simulink model "buck"  (R2023b)
settings: Solver=VariableStepAuto  StartTime=0.0  StopTime=0.05  FixedStep=60e-6  MaxStep=1e-6  RelTol=1e-3
undefined symbols (not defined in the file): C, L, R, R1, R2, R3, R4, R_in, Vi
settings Model: Creator=Jackson  LastModifiedBy=Jackson

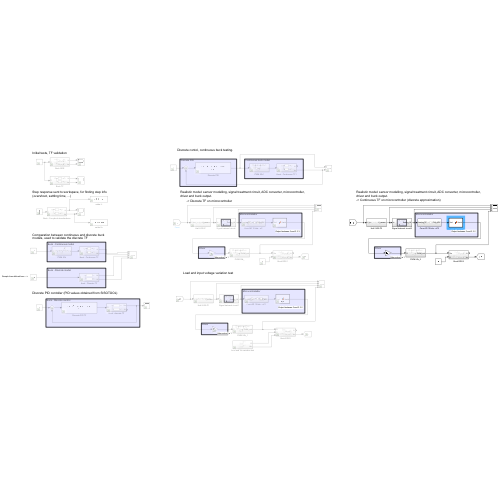
[thumbnail: Simulink's stored preview of the top-level diagram]
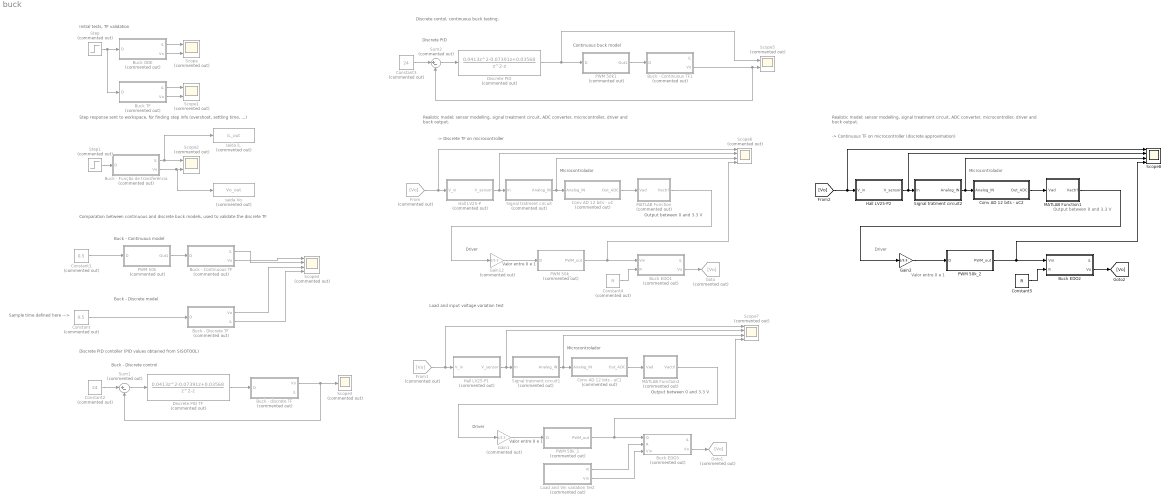
== system buck ==
  note: -> Discrete TF on microcontroller
  note: Initial tests, TF validation
  note: Output between 0 and 3.3 V
  note: Buck - Discrete control
  note: Buck - Discrete model
  note: Buck - Continuous model
  note: Discrete PID
  note: Continuous buck model
  note: Driver
  note: Microcontrolador
  note: Valor entre 0 e 1
  note: Step response sent to workspace, for finding step info (overshoot, settling time, ...)
  note: Comparation between continuous and discrete buck models, used to validate the discrete TF
  note: Sample time defined here --->
  note: Discrete PID contoller (PID values obtained from SISOTOOL)
  note: Discrete contol, continuous buck testing.
  note: Realistic model: sensor modelling, signal treatment circuit, ADC converter, microcontroller, driver and buck output.
  note: Microcontrolador
  note: Valor entre 0 e 1
  note: Driver
  note: Load and input voltage variation test
  note: Output between 0 and 3.3 V
  note: Microcontrolador
  note: Valor entre 0 e 1
  note: Driver
  note: Realistic model: sensor modelling, signal treatment circuit, ADC converter, microcontroller, driver and buck output.
  note: Output between 0 and 3.3 V
  note: -> Continuous TF on microcontroller (discrete approximation)
  Buck - Continuous TF : Subsystem  Commented=on
  Buck - Continuous TF1 : Subsystem  Commented=on
  Buck - Discrete TF : Subsystem  Commented=on
  Buck - Função de transferência : Subsystem  Commented=on
  Buck - discrete TF : Subsystem  Commented=on
  Buck EDO1 : Subsystem  Commented=on
  Buck EDO2 : Subsystem
  Buck EDO3 : Subsystem  Commented=on
  Buck ODE : Subsystem  Commented=on
  Buck TF : Subsystem  Commented=on
  Constant : Constant  Commented=on  Value=0.5  SampleTime=60e-6
  Constant1 : Constant  Commented=on  Value=0.5
  Constant2 : Constant  Commented=on  Value=24  SampleTime=60e-6
  Constant3 : Constant  Commented=on  Value=24  SampleTime=60e-6
  Constant4 : Constant  Commented=on  Value=R  SampleTime=60e-6
  Constant5 : Constant  Value=R  SampleTime=60e-6
  Conv AD 12 bits - uC : Subsystem  Commented=on
  Conv AD 12 bits - uC1 : Subsystem  Commented=on
  Conv AD 12 bits - uC2 : Subsystem
  Discrete PID : DiscreteTransferFcn  Commented=on  Numerator=[0.0413 -0.07391 0.03568]  Denominator=[1 -1 0]
  Discrete PID TF : DiscreteTransferFcn  Commented=on  Numerator=[0.0413 -0.07391 0.03568]  Denominator=[1 -1 0]
  From : From  Commented=on  GotoTag=Vo
  From1 : From  Commented=on  GotoTag=Vo
  Gain1 : Gain  Commented=on  Gain=1/3.3
  Gain12 : Gain  Commented=on  Gain=1/3.3
  Gain2 : Gain  Gain=1/3.3
  Goto : Goto  Commented=on  GotoTag=Vo
  Goto1 : Goto  Commented=on  GotoTag=Vo
  Hall LV25-P : Subsystem  Commented=on
  Hall LV25-P1 : Subsystem  Commented=on
  Hall LV25-P2 : Subsystem
  Load and Vin variation test : Subsystem  Commented=on
  MATLAB Function : MATLAB Function  Commented=on  TreatAsAtomicUnit=on
  MATLAB Function1 : MATLAB Function  TreatAsAtomicUnit=on
  MATLAB Function2 : MATLAB Function  Commented=on  TreatAsAtomicUnit=on
  PWM 50k : Subsystem  Commented=on
  PWM 50k1 : Subsystem  Commented=on
  PWM 50k_ : Subsystem  Commented=on
  PWM 50k_1 : Subsystem  Commented=on
  PWM 50k_2 : Subsystem
  Scope{,1..2,5} (4 alike) : Scope  Commented=on  NumInputPorts=2
  Scope3 : Scope  Commented=on
  Scope4 : Scope  Commented=on  NumInputPorts=4
  Scope6 : Scope  Commented=on  NumInputPorts=4
  Scope7 : Scope  Commented=on  NumInputPorts=4
  Scope8 : Scope  NumInputPorts=4
  Signal tratment circuit : Subsystem  Commented=on
  Signal tratment circuit1 : Subsystem  Commented=on
  Signal tratment circuit2 : Subsystem
  Step : Step  Commented=on  Time=0  SampleTime=0
  Step1 : Step  Commented=on  Time=0  SampleTime=0
  Sum1 : Sum  Commented=on  Inputs=|+-
  Sum2 : Sum  Commented=on  Inputs=|+-
  saída Vo : ToWorkspace  Commented=on  VariableName=Vo_out  SaveFormat=Timeseries  SampleTime=-1
  saída iL : ToWorkspace  Commented=on  VariableName=iL_out  SaveFormat=Timeseries  SampleTime=-1
  wires:
  Step/1 -> Buck TF/1(D), Buck ODE/1(D)
  Buck ODE/1(iL) -> Scope/1
  Buck ODE/2(Vo) -> Scope/2
  Buck TF/2(Vo) -> Scope1/2
  Buck TF/1(iL) -> Scope1/1
  Buck - Função de transferência/2(Vo) -> saída Vo/1, Scope2/2
  Buck - Função de transferência/1(iL) -> saída iL/1, Scope2/1
  Step1/1 -> Buck - Função de transferência/1(D)
  Buck - Continuous TF/2(Vo) -> Scope4/1
  PWM 50k/1(Out1) -> Buck - Continuous TF/1(D)
  Constant1/1 -> PWM 50k/1(D)
  Buck - Discrete TF/1(Vo) -> Scope4/3
  Buck - Discrete TF/2(iL) -> Scope4/4
  Constant/1 -> Buck - Discrete TF/1(D)
  Buck - Continuous TF/1(iL) -> Scope4/2
  Sum1/1 -> Discrete PID TF/1
  Buck - discrete TF/1(Vo) -> Sum1/2, Scope3/1
  Constant2/1 -> Sum1/1
  Discrete PID TF/1 -> Buck - discrete TF/1(D)
  Sum2/1 -> Discrete PID/1
  Buck - Continuous TF1/2(Vo) -> Sum2/2, Scope5/2
  Constant3/1 -> Sum2/1
  Discrete PID/1 -> PWM 50k1/1(D), Scope5/1
  PWM 50k1/1(Out1) -> Buck - Continuous TF1/1(D)
  Constant4/1 -> Buck EDO1/2(R)
  Hall LV25-P/1(V_sensor) -> Scope6/2, Signal tratment circuit/1(In)
  Signal tratment circuit/1(Analog_IN) -> Scope6/3, Conv AD 12 bits - uC/1(Analog_IN)
  Conv AD 12 bits - uC/1(Out_ADC) -> MATLAB Function/1(Vad)
  MATLAB Function/1(Vactrl) -> Gain12/1
  Gain12/1 -> PWM 50k_/1(D)
  PWM 50k_/1(PWM_out) -> Scope6/4, Buck EDO1/1(Vin)
  Buck EDO1/2(Vo) -> Goto/1
  From/1 -> Scope6/1, Hall LV25-P/1(V_in)
  Hall LV25-P1/1(V_sensor) -> Scope7/2, Signal tratment circuit1/1(In)
  PWM 50k_1/1(PWM_out) -> Scope7/4, Buck EDO3/1(D)
  Gain1/1 -> PWM 50k_1/1(D)
  Conv AD 12 bits - uC1/1(Out_ADC) -> MATLAB Function2/1(Vad)
  Signal tratment circuit1/1(Analog_IN) -> Scope7/3, Conv AD 12 bits - uC1/1(Analog_IN)
  MATLAB Function2/1(Vactrl) -> Gain1/1
  From1/1 -> Scope7/1, Hall LV25-P1/1(V_in)
  Buck EDO3/2(Vo) -> Goto1/1
  Load and Vin variation test/1(R) -> Buck EDO3/2(R)
  Load and Vin variation test/2(Vin) -> Buck EDO3/3(Vin)
  Hall LV25-P2/1(V_sensor) -> Scope8/2, Signal tratment circuit2/1(In)
  PWM 50k_2/1(PWM_out) -> Scope8/4, Buck EDO2/1(Vin)
  Gain2/1 -> PWM 50k_2/1(D)
  Conv AD 12 bits - uC2/1(Out_ADC) -> MATLAB Function1/1(Vad)
  Signal tratment circuit2/1(Analog_IN) -> Scope8/3, Conv AD 12 bits - uC2/1(Analog_IN)
  MATLAB Function1/1(Vactrl) -> Gain2/1
  [Vo] -> Scope8/1, Hall LV25-P2/1(V_in)
  Buck EDO2/2(Vo) -> [Vo]
  Constant5/1 -> Buck EDO2/2(R)

== system buck/Buck - Continuous TF ==
  D : Inport
  Gi : TransferFcn  Numerator=[Vi*C Vi/R]  Denominator=[L*C L/R 1]
  Gv : TransferFcn  Numerator=[Vi/(L*C)]  Denominator=[1 1/(R*C) 1/(L*C)]
  iL : Outport
  Vo : Outport  Port=2
  wires:
  Gv/1 -> Vo/1
  Gi/1 -> iL/1
  D/1 -> Gv/1, Gi/1

== system buck/Buck - Continuous TF1 ==
  D : Inport
  Gi : TransferFcn  Numerator=[Vi*C Vi/R]  Denominator=[L*C L/R 1]
  Gv : TransferFcn  Numerator=[Vi/(L*C)]  Denominator=[1 1/(R*C) 1/(L*C)]
  iL : Outport
  Vo : Outport  Port=2
  wires:
  Gv/1 -> Vo/1
  Gi/1 -> iL/1
  D/1 -> Gv/1, Gi/1

== system buck/Buck - Discrete TF ==
  D : Inport
  Gi(z)1 : DiscreteTransferFcn  Numerator=[1.341 -1.051]  Denominator=[1 -1.629 0.7866]
  Gv(z) : DiscreteTransferFcn  Numerator=[3.772 3.48]  Denominator=[1 -1.629 0.7866]
  Vo : Outport
  iL : Outport  Port=2
  wires:
  Gv(z)/1 -> Vo/1
  D/1 -> Gi(z)1/1, Gv(z)/1
  Gi(z)1/1 -> iL/1

== system buck/Buck - Função de transferência ==
  D : Inport
  Gi : TransferFcn  Numerator=[Vi*C Vi/R]  Denominator=[L*C L/R 1]
  Gv : TransferFcn  Numerator=[Vi/(L*C)]  Denominator=[1 1/(R*C) 1/(L*C)]
  iL : Outport
  Vo : Outport  Port=2
  wires:
  Gv/1 -> Vo/1
  Gi/1 -> iL/1
  D/1 -> Gv/1, Gi/1

== system buck/Buck - discrete TF ==
  D : Inport
  Gi(z)1 : DiscreteTransferFcn  Numerator=[1.341 -1.051]  Denominator=[1 -1.629 0.7866]
  Gv(z) : DiscreteTransferFcn  Numerator=[3.772 3.48]  Denominator=[1 -1.629 0.7866]
  Vo : Outport
  iL : Outport  Port=2
  wires:
  Gv(z)/1 -> Vo/1
  D/1 -> Gi(z)1/1, Gv(z)/1
  Gi(z)1/1 -> iL/1

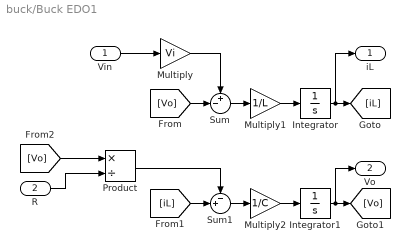
== system buck/Buck EDO1 ==
  Vin : Inport
  R : Inport  Port=2
  Integrator : Integrator
  Integrator1 : Integrator
  Multiply : Gain  Gain=Vi
  Multiply1 : Gain  Gain=1/L
  Multiply2 : Gain  Gain=1/C
  Product : Product  Inputs=*/
  Sum : Sum  Inputs=+-|
  Sum1 : Sum  Inputs=-+|
  iL : Outport
  Vo : Outport  Port=2
  wires:
  [Vo] -> Product/1
  Multiply2/1 -> Integrator1/1
  Sum1/1 -> Multiply2/1
  Integrator1/1 -> Vo/1, [Vo]
  Integrator/1 -> iL/1, [iL]
  [iL] -> Sum1/2
  [Vo] -> Sum/2
  Sum/1 -> Multiply1/1
  Multiply1/1 -> Integrator/1
  Vin/1 -> Multiply/1
  Multiply/1 -> Sum/1
  R/1 -> Product/2
  Product/1 -> Sum1/1

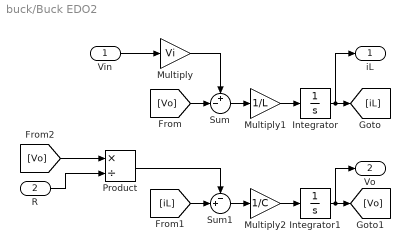
== system buck/Buck EDO2 ==
  Vin : Inport
  R : Inport  Port=2
  Integrator : Integrator
  Integrator1 : Integrator
  Multiply : Gain  Gain=Vi
  Multiply1 : Gain  Gain=1/L
  Multiply2 : Gain  Gain=1/C
  Product : Product  Inputs=*/
  Sum : Sum  Inputs=+-|
  Sum1 : Sum  Inputs=-+|
  iL : Outport
  Vo : Outport  Port=2
  wires:
  [Vo] -> Product/1
  Multiply2/1 -> Integrator1/1
  Sum1/1 -> Multiply2/1
  Integrator1/1 -> Vo/1, [Vo]
  Integrator/1 -> iL/1, [iL]
  [iL] -> Sum1/2
  [Vo] -> Sum/2
  Sum/1 -> Multiply1/1
  Multiply1/1 -> Integrator/1
  Vin/1 -> Multiply/1
  Multiply/1 -> Sum/1
  R/1 -> Product/2
  Product/1 -> Sum1/1

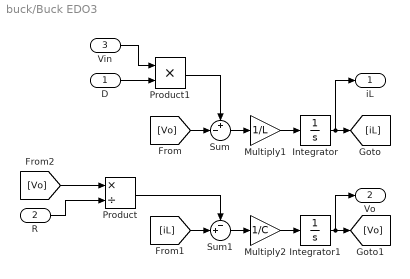
== system buck/Buck EDO3 ==
  D : Inport
  R : Inport  Port=2
  Vin : Inport  Port=3
  Integrator : Integrator
  Integrator1 : Integrator
  Multiply1 : Gain  Gain=1/L
  Multiply2 : Gain  Gain=1/C
  Product : Product  Inputs=*/
  Product1 : Product
  Sum : Sum  Inputs=+-|
  Sum1 : Sum  Inputs=-+|
  iL : Outport
  Vo : Outport  Port=2
  wires:
  [Vo] -> Product/1
  Multiply2/1 -> Integrator1/1
  Sum1/1 -> Multiply2/1
  Integrator1/1 -> Vo/1, [Vo]
  Integrator/1 -> iL/1, [iL]
  [iL] -> Sum1/2
  [Vo] -> Sum/2
  Sum/1 -> Multiply1/1
  Multiply1/1 -> Integrator/1
  D/1 -> Product1/2
  Product1/1 -> Sum/1
  R/1 -> Product/2
  Product/1 -> Sum1/1
  Vin/1 -> Product1/1

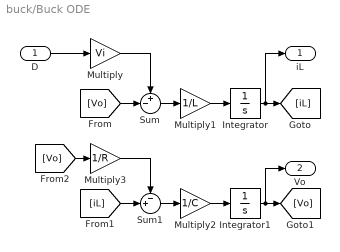
== system buck/Buck ODE ==
  D : Inport
  Integrator : Integrator
  Integrator1 : Integrator
  Multiply : Gain  Gain=Vi
  Multiply1 : Gain  Gain=1/L
  Multiply2 : Gain  Gain=1/C
  Multiply3 : Gain  Gain=1/R
  Sum : Sum  Inputs=+-|
  Sum1 : Sum  Inputs=-+|
  iL : Outport
  Vo : Outport  Port=2
  wires:
  Multiply3/1 -> Sum1/1
  [Vo] -> Multiply3/1
  Multiply2/1 -> Integrator1/1
  Sum1/1 -> Multiply2/1
  Integrator1/1 -> Vo/1, [Vo]
  Integrator/1 -> iL/1, [iL]
  [iL] -> Sum1/2
  [Vo] -> Sum/2
  Sum/1 -> Multiply1/1
  Multiply1/1 -> Integrator/1
  D/1 -> Multiply/1
  Multiply/1 -> Sum/1

== system buck/Buck TF ==
  D : Inport
  Gi : TransferFcn  Numerator=[Vi*C Vi/R]  Denominator=[L*C L/R 1]
  Gv : TransferFcn  Numerator=[Vi/(L*C)]  Denominator=[1 1/(R*C) 1/(L*C)]
  iL : Outport
  Vo : Outport  Port=2
  wires:
  Gv/1 -> Vo/1
  Gi/1 -> iL/1
  D/1 -> Gv/1, Gi/1

== system buck/Conv AD 12 bits - uC ==
  Analog_IN : Inport
  Gain11 : Gain  Gain=4095/3.3
  Quantizer : Quantizer  QuantizationInterval=1
  Rate Transition1 : RateTransition  OutPortSampleTime=Ts
  Out_ADC : Outport
  wires:
  Quantizer/1 -> Rate Transition1/1
  Gain11/1 -> Quantizer/1
  Rate Transition1/1 -> Out_ADC/1
  Analog_IN/1 -> Gain11/1

== system buck/Conv AD 12 bits - uC1 ==
  Analog_IN : Inport
  Gain11 : Gain  Gain=4095/3.3
  Quantizer : Quantizer  QuantizationInterval=1
  Rate Transition1 : RateTransition  OutPortSampleTime=Ts
  Out_ADC : Outport
  wires:
  Quantizer/1 -> Rate Transition1/1
  Gain11/1 -> Quantizer/1
  Rate Transition1/1 -> Out_ADC/1
  Analog_IN/1 -> Gain11/1

== system buck/Conv AD 12 bits - uC2 ==
  Analog_IN : Inport
  Gain11 : Gain  Gain=4095/3.3
  Quantizer : Quantizer  QuantizationInterval=1
  Rate Transition1 : RateTransition  OutPortSampleTime=Ts
  Out_ADC : Outport
  wires:
  Quantizer/1 -> Rate Transition1/1
  Gain11/1 -> Quantizer/1
  Rate Transition1/1 -> Out_ADC/1
  Analog_IN/1 -> Gain11/1

== system buck/Hall LV25-P ==
  note: I_p
  note: I_s
  note: V_o
  V_in : Inport
  Ganho resist. entrada : Gain  Gain=1/R_in
  Ganho trafo : Gain  Gain=2.5
  ganho R_med : Gain  Gain=100
  V_sensor : Outport
  wires:
  V_in/1 -> Ganho resist. entrada/1
  Ganho resist. entrada/1 -> Ganho trafo/1
  Ganho trafo/1 -> ganho R_med/1
  ganho R_med/1 -> V_sensor/1

== system buck/Hall LV25-P1 ==
  note: I_p
  note: I_s
  note: V_o
  V_in : Inport
  Ganho resist. entrada : Gain  Gain=1/R_in
  Ganho trafo : Gain  Gain=2.5
  ganho R_med : Gain  Gain=100
  V_sensor : Outport
  wires:
  V_in/1 -> Ganho resist. entrada/1
  Ganho resist. entrada/1 -> Ganho trafo/1
  Ganho trafo/1 -> ganho R_med/1
  ganho R_med/1 -> V_sensor/1

== system buck/Hall LV25-P2 ==
  note: I_p
  note: I_s
  note: V_o
  V_in : Inport
  Ganho resist. entrada : Gain  Gain=1/R_in
  Ganho trafo : Gain  Gain=2.5
  ganho R_med : Gain  Gain=100
  V_sensor : Outport
  wires:
  V_in/1 -> Ganho resist. entrada/1
  Ganho resist. entrada/1 -> Ganho trafo/1
  Ganho trafo/1 -> ganho R_med/1
  ganho R_med/1 -> V_sensor/1

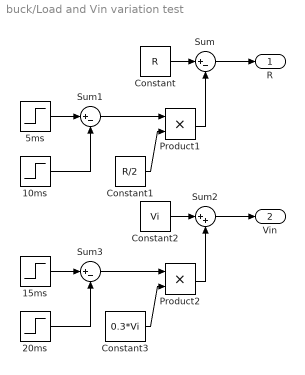
== system buck/Load and Vin variation test ==
  10ms : Step  Time=0.01  SampleTime=0
  15ms : Step  Time=0.015  SampleTime=0
  20ms : Step  Time=0.02  SampleTime=0
  5ms : Step  Time=0.005  SampleTime=0
  Constant : Constant  Value=R
  Constant1 : Constant  Value=R/2
  Constant2 : Constant  Value=Vi
  Constant3 : Constant  Value=0.3*Vi
  Product1 : Product
  Product2 : Product
  Sum : Sum  Inputs=|+-
  Sum1 : Sum  Inputs=|+-
  Sum2 : Sum  Inputs=|++
  Sum3 : Sum  Inputs=|+-
  R : Outport
  Vin : Outport  Port=2
  wires:
  Constant/1 -> Sum/1
  Sum/1 -> R/1
  5ms/1 -> Sum1/1
  10ms/1 -> Sum1/2
  Sum1/1 -> Product1/1
  Product1/1 -> Sum/2
  Constant1/1 -> Product1/2
  Sum3/1 -> Product2/1
  Sum2/1 -> Vin/1
  15ms/1 -> Sum3/1
  Product2/1 -> Sum2/2
  Constant2/1 -> Sum2/1
  Constant3/1 -> Product2/2
  20ms/1 -> Sum3/2

== system buck/PWM 50k ==
  D : Inport
  Constant : Constant
  Gain : Gain  Gain=0.5
  Relay : Relay
  Sawtooth Generator : SignalGenerator  WaveForm=sawtooth  Frequency=50000
  Scope : Scope  NumInputPorts=3
  Sum : Sum  Inputs=|++
  Sum1 : Sum  Inputs=|+-
  Out1 : Outport
  wires:
  Sawtooth Generator/1 -> Sum/2
  Constant/1 -> Sum/1
  Sum/1 -> Gain/1
  Relay/1 -> Out1/1
  Gain/1 -> Sum1/1
  Sum1/1 -> Scope/3, Relay/1
  D/1 -> Sum1/2

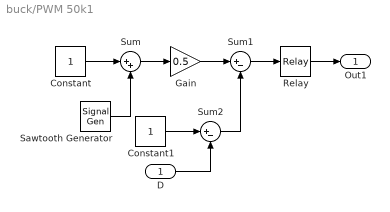
== system buck/PWM 50k1 ==
  D : Inport
  Constant : Constant
  Constant1 : Constant
  Gain : Gain  Gain=0.5
  Relay : Relay
  Sawtooth Generator : SignalGenerator  WaveForm=sawtooth  Frequency=50000
  Sum : Sum  Inputs=|++
  Sum1 : Sum  Inputs=|+-
  Sum2 : Sum  Inputs=|+-
  Out1 : Outport
  wires:
  Sawtooth Generator/1 -> Sum/2
  Constant/1 -> Sum/1
  Sum/1 -> Gain/1
  Relay/1 -> Out1/1
  Gain/1 -> Sum1/1
  Sum1/1 -> Relay/1
  Sum2/1 -> Sum1/2
  Constant1/1 -> Sum2/1
  D/1 -> Sum2/2

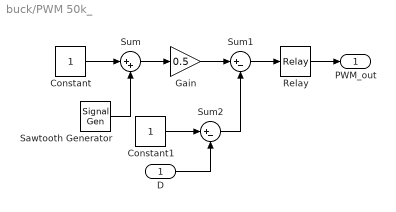
== system buck/PWM 50k_ ==
  D : Inport
  Constant : Constant
  Constant1 : Constant
  Gain : Gain  Gain=0.5
  Relay : Relay
  Sawtooth Generator : SignalGenerator  WaveForm=sawtooth  Frequency=50000
  Sum : Sum  Inputs=|++
  Sum1 : Sum  Inputs=|+-
  Sum2 : Sum  Inputs=|+-
  PWM_out : Outport
  wires:
  Sawtooth Generator/1 -> Sum/2
  Constant/1 -> Sum/1
  Sum/1 -> Gain/1
  Relay/1 -> PWM_out/1
  Gain/1 -> Sum1/1
  Sum1/1 -> Relay/1
  Sum2/1 -> Sum1/2
  Constant1/1 -> Sum2/1
  D/1 -> Sum2/2

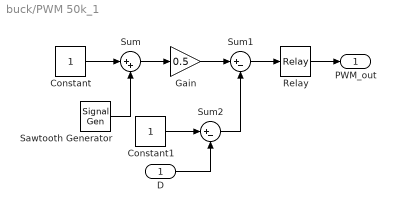
== system buck/PWM 50k_1 ==
  D : Inport
  Constant : Constant
  Constant1 : Constant
  Gain : Gain  Gain=0.5
  Relay : Relay
  Sawtooth Generator : SignalGenerator  WaveForm=sawtooth  Frequency=50000
  Sum : Sum  Inputs=|++
  Sum1 : Sum  Inputs=|+-
  Sum2 : Sum  Inputs=|+-
  PWM_out : Outport
  wires:
  Sawtooth Generator/1 -> Sum/2
  Constant/1 -> Sum/1
  Sum/1 -> Gain/1
  Relay/1 -> PWM_out/1
  Gain/1 -> Sum1/1
  Sum1/1 -> Relay/1
  Sum2/1 -> Sum1/2
  Constant1/1 -> Sum2/1
  D/1 -> Sum2/2

== system buck/PWM 50k_2 ==
  D : Inport
  Constant : Constant
  Constant1 : Constant
  Gain : Gain  Gain=0.5
  Relay : Relay
  Sawtooth Generator : SignalGenerator  WaveForm=sawtooth  Frequency=50000
  Sum : Sum  Inputs=|++
  Sum1 : Sum  Inputs=|+-
  Sum2 : Sum  Inputs=|+-
  PWM_out : Outport
  wires:
  Sawtooth Generator/1 -> Sum/2
  Constant/1 -> Sum/1
  Sum/1 -> Gain/1
  Relay/1 -> PWM_out/1
  Gain/1 -> Sum1/1
  Sum1/1 -> Relay/1
  Sum2/1 -> Sum1/2
  Constant1/1 -> Sum2/1
  D/1 -> Sum2/2

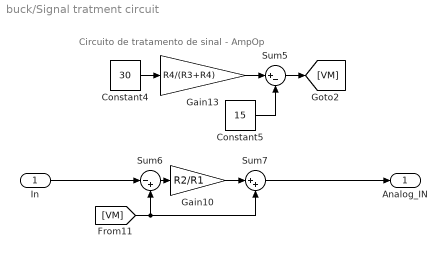
== system buck/Signal tratment circuit ==
  note: Circuito de tratamento de sinal - AmpOp
  In : Inport
  Constant4 : Constant  Value=30
  Constant5 : Constant  Value=15
  Gain10 : Gain  Gain=R2/R1
  Gain13 : Gain  Gain=R4/(R3+R4)
  Sum5 : Sum  Inputs=|+-
  Sum6 : Sum  Inputs=|-+
  Sum7 : Sum  Inputs=|++
  Analog_IN : Outport
  wires:
  Sum7/1 -> Analog_IN/1
  Sum6/1 -> Gain10/1
  [VM] -> Sum7/2, Sum6/2
  Constant5/1 -> Sum5/2
  Constant4/1 -> Gain13/1
  Gain13/1 -> Sum5/1
  Gain10/1 -> Sum7/1
  Sum5/1 -> [VM]
  In/1 -> Sum6/1

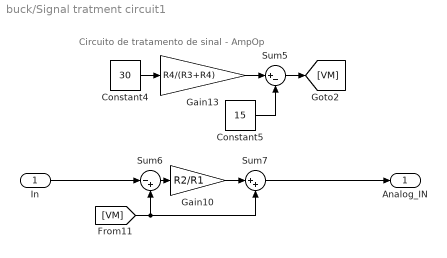
== system buck/Signal tratment circuit1 ==
  note: Circuito de tratamento de sinal - AmpOp
  In : Inport
  Constant4 : Constant  Value=30
  Constant5 : Constant  Value=15
  Gain10 : Gain  Gain=R2/R1
  Gain13 : Gain  Gain=R4/(R3+R4)
  Sum5 : Sum  Inputs=|+-
  Sum6 : Sum  Inputs=|-+
  Sum7 : Sum  Inputs=|++
  Analog_IN : Outport
  wires:
  Sum7/1 -> Analog_IN/1
  Sum6/1 -> Gain10/1
  [VM] -> Sum7/2, Sum6/2
  Constant5/1 -> Sum5/2
  Constant4/1 -> Gain13/1
  Gain13/1 -> Sum5/1
  Gain10/1 -> Sum7/1
  Sum5/1 -> [VM]
  In/1 -> Sum6/1

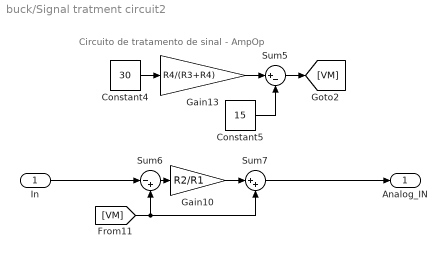
== system buck/Signal tratment circuit2 ==
  note: Circuito de tratamento de sinal - AmpOp
  In : Inport
  Constant4 : Constant  Value=30
  Constant5 : Constant  Value=15
  Gain10 : Gain  Gain=R2/R1
  Gain13 : Gain  Gain=R4/(R3+R4)
  Sum5 : Sum  Inputs=|+-
  Sum6 : Sum  Inputs=|-+
  Sum7 : Sum  Inputs=|++
  Analog_IN : Outport
  wires:
  Sum7/1 -> Analog_IN/1
  Sum6/1 -> Gain10/1
  [VM] -> Sum7/2, Sum6/2
  Constant5/1 -> Sum5/2
  Constant4/1 -> Gain13/1
  Gain13/1 -> Sum5/1
  Gain10/1 -> Sum7/1
  Sum5/1 -> [VM]
  In/1 -> Sum6/1

== matlab function buck/MATLAB Function ==
  data: Vad input; Vactrl output
function Vactrl = fcn(Vad)

% Valor de Vo desejado, programado no uC
Vo_ref = 24

R_in = 10000

% Aproximação comercial
R1 = 10e3
R2 = 10800
R3 = 82000
R4 = 100e3

% Mapeamento reverso
V2 = 3.3 * Vad / 4095
Vm = 30*(R4/(R3+R4))-15
V1 = R1/R2*(Vm-V2)+Vm
Vo = V1 * R_in / 250

e = Vo_ref - Vo

persistent u_1;
persistent e_1;
persistent e_2;
if isempty(u_1)
   u_1 = cast(0, 'like', Vo);
end
if isempty(e_1)
    e_1 = cast(0, 'like', e);
end
if isempty(e_2)
    e_2 = cast(0, 'like', e);
end

Vactrl = u_1 + 0.0413 * e - 0.0739 * e_1 + 0.0357 * e_2;

% Deve sair valor de 0 a 5 V para o PWM.
if (Vactrl < 0)
    Vactrl = 0
end
if (Vactrl > 3.3)
    Vactrl = 3.3
end

 % store the current input
 u_1 = Vactrl;
 e_1 = e;
 e_2 = e_1;

== matlab function buck/MATLAB Function2 ==
  data: Vad input; Vactrl output
function Vactrl = fcn(Vad)

% Valor de Vo desejado, programado no uC
Vo_ref = 24

R_in = 10000

% Aproximação comercial
R1 = 10e3
R2 = 10800
R3 = 82000
R4 = 100e3

% Mapeamento reverso
V2 = 3.3 * Vad / 4095
Vm = 30*(R4/(R3+R4))-15
V1 = R1/R2*(Vm-V2)+Vm
Vo = V1 * R_in / 250

e = Vo_ref - Vo

persistent u_1;
persistent e_1;
persistent e_2;
if isempty(u_1)
   u_1 = cast(0, 'like', Vo);
end
if isempty(e_1)
    e_1 = cast(0, 'like', e);
end
if isempty(e_2)
    e_2 = cast(0, 'like', e);
end

Vactrl = u_1 + 0.0413 * e - 0.0739 * e_1 + 0.0357 * e_2;

% Deve sair valor de 0 a 5 V para o PWM.
if (Vactrl < 0)
    Vactrl = 0
end
if (Vactrl > 3.3)
    Vactrl = 3.3
end

 % store the current input
 u_1 = Vactrl;
 e_1 = e;
 e_2 = e_1;

== matlab function buck/MATLAB Function1 ==
  data: Vad input; Vactrl output
function Vactrl = fcn(Vad)

% Valor de Vo desejado, programado no uC
Vo_ref = 24

R_in = 10000

% Aproximação comercial
R1 = 10e3
R2 = 10800
R3 = 82000
R4 = 100e3

% Mapeamento reverso
V2 = 3.3 * Vad / 4095
Vm = 30*(R4/(R3+R4))-15
V1 = R1/R2*(Vm-V2)+Vm
Vo = V1 * R_in / 250

e = Vo_ref - Vo

persistent u_1;
persistent e_1;
persistent e_2;
persistent Ik_1;

if isempty(u_1)
   u_1 = cast(0, 'like', Vo);
end
if isempty(e_1)
    e_1 = cast(0, 'like', e);
end
if isempty(e_2)
    e_2 = cast(0, 'like', e);
end

if isempty(Ik_1)
    Ik_1 = 0;
end

% Ganhos do controlador PID contínuo discretizado
kp = 0.013;
kd = 3.24e-6;
ki = 100;

%Cálculo das aproximações derivada e integral (controle contínuo)----------
Ts = 6e-5;
dk = (e - e_1)/Ts;
Ak = (e + e_1)/2*Ts
Ik = Ik_1 + Ak;

%Cálculo do esforço de controle--------------------------------------------
Vactrl = kp*e + ki*Ik + kd*dk; %Controle contínuo discretizado
%Vactrl = u_1 + 0.0413 * e - 0.0739 * e_1 + 0.0357 * e_2; %Controle discreto

% Deve sair valor de 0 a 3.3 V para o PWM.
if (Vactrl < 0)
    Vactrl = 0
end
if (Vactrl > 3.3)
    Vactrl = 3.3
end

 % store the current input
 u_1 = Vactrl;
 e_1 = e;
 e_2 = e_1;
 Ik_1 = Ik;
